simulink model "lab08q2"  (Simulink 7.1)
settings: Solver=ode45  StartTime=0.0  StopTime=1  RelTol=1e-3
InitFcn:
  | C1= 0.00000025;
  | C2= 0.00000025;
  | k= 1;
  | R1=40000;
  | R2=60000;
  | 
  | A = [((-1/(R1*C1))-(1/(R2*C1))) ((1+k)*(1/(R1*C1))+k*(1/(R2*C1)));(-1/(R2*C2)) (1/(R2*C2))*k]
  | 
  | B = [-(1/(R1*C1));0]
  | 
  | C = [0 (1+k);1 0;0 1]
  | 
  | D = [0;0;0]
settings Model: Creator=ALUNO  LastModifiedBy=ALUNO
settings DebuggingCC: SaveWithParameterizedLinksMsg=none

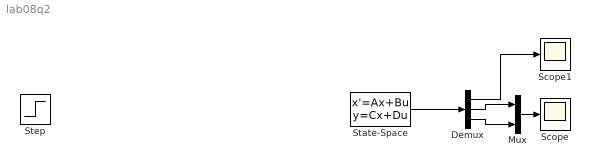
== system lab08q2 ==
  Demux : Demux  Outputs=3
  Mux : Mux  Inputs=2
  Scope : Scope
  Scope1 : Scope
      settings: TimeRange=1  YMin=0  YMax=1
  State-Space : StateSpace  A=A  B=B  C=C  D=D
  Step : Step  Time=0  SampleTime=0
  wires:
  State-Space/1 -> Demux/1
  Mux/1 -> Scope/1
  Demux/1 -> Scope1/1
  Demux/2 -> Mux/1
  Demux/3 -> Mux/2
